simulink model "thomas_sim"  (R2021a)
settings: Solver=FixedStepAuto  StartTime=0.0  StopTime=500  FixedStep=0.001  RelTol=1e-3
values from neighbouring files (symbols this model uses):
  x0 = [-0.1 0.5 -0.6]    [Attractors.m]    (also in thomas_system_phasediagram.m = [ 5;2.7;0 ])
settings Model: Creator=toure  LastModifiedBy=toure

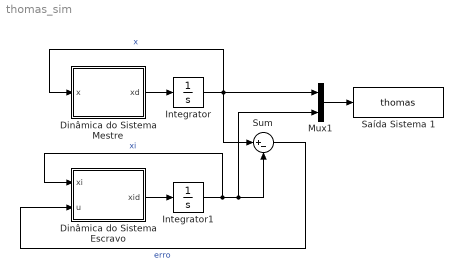
== system thomas_sim ==
  Dinâmica do Sistema Escravo : MATLAB Function  TreatAsAtomicUnit=on
  Dinâmica do Sistema Mestre : MATLAB Function  TreatAsAtomicUnit=on
  Integrator : Integrator  InitialCondition=x0
  Integrator1 : Integrator  InitialCondition=37.54*x0
  Mux1 : Mux  Inputs=2
  Saída Sistema 1 : ToWorkspace  VariableName=thomas  SaveFormat=Timeseries  SampleTime=-1
      settings: Save2DSignal=2-D array (concatenate along first dimension)
  Sum : Sum  Inputs=|+-
  wires:
  Dinâmica do Sistema Mestre/1(xd) -> Integrator/1
  Integrator/1 -> Dinâmica do Sistema Mestre/1(x), Mux1/1, Sum/1  "x"
  Integrator1/1 -> Mux1/2, Sum/2, Dinâmica do Sistema Escravo/1(xi)  "xi"
  Dinâmica do Sistema Escravo/1(xid) -> Integrator1/1
  Sum/1 -> Dinâmica do Sistema Escravo/2(u)  "erro"
  Mux1/1 -> Saída Sistema 1/1

== matlab function thomas_sim/Dinâmica do Sistema Mestre ==
  data: x input; xd output; b parameter
function xd = fcn(x,b)

xd = [sin(x(2)) + b*x(1)
      sin(x(3)) + b*x(2)
      sin(x(1)) + b*x(3)];
end

== matlab function thomas_sim/Dinâmica do Sistema Escravo ==
  data: xi input; u input; xid output; b parameter
function xid = fcn(xi,u,b)

xid = [sin(xi(2)) + b*xi(1) + u(1)
       sin(xi(3)) + b*xi(2) + u(2)
       sin(xi(1)) + b*xi(3) + u(3)];
end
